simulink model "obsvsimulink"  (R2018b)
settings: Solver=VariableStepAuto  StartTime=0.0  StopTime=10  RelTol=1e-3
values from neighbouring files (symbols this model uses):
  A = [0 1 0 0 ... (first row only)    [kalman.m]    (also in lqr_controller.m; lqr_observare.m; state_space.m)
  B = [0 ... (first row only)    [kalman.m]    (also in lqr_controller.m; lqr_observare.m; state_space.m)
  C = [1 0 0 0;]    [kalman.m]    (also in lqr_controller.m = [1 0 0 0; lqr_observare.m = [1 0 0 0; state_space.m = [1 0 0 0)
  K_d = lqr(A,B,Q,R)    [lqr_observare.m]
  L_o = (place(A',C',E))'    [lqr_observare.m]
settings Model: Creator=SAFARBALI  LastModifiedBy=888
settings SFSimCC: SimUseLocalCustomCode=off
settings RTWCC: RTWUseLocalCustomCode=off
settings CodeAppCC: StateflowObjectComments=on

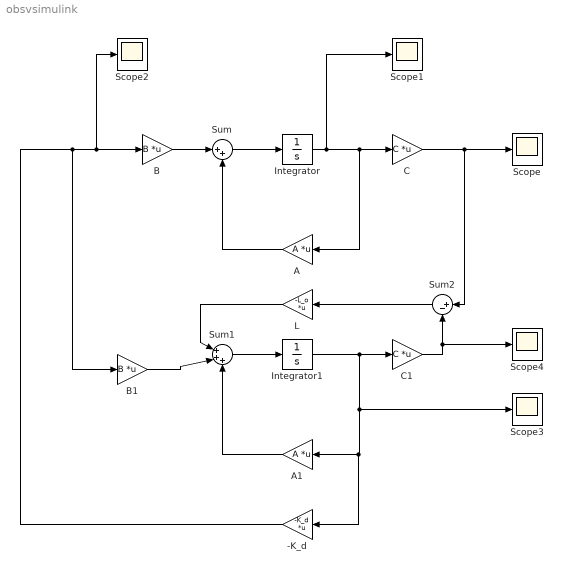
== system obsvsimulink ==
  -K_d : Gain  Gain=-K_d  Multiplication=Matrix(K*u)
  A : Gain  Gain=A  Multiplication=Matrix(K*u)
  A1 : Gain  Gain=A  Multiplication=Matrix(K*u)
  B : Gain  Gain=B  Multiplication=Matrix(K*u)
  B1 : Gain  Gain=B  Multiplication=Matrix(K*u)
  C : Gain  Gain=C  Multiplication=Matrix(K*u)
  C1 : Gain  Gain=C  Multiplication=Matrix(K*u)
  Integrator : Integrator  InitialCondition=[0;5;0;0]
  Integrator1 : Integrator  InitialCondition=[0;5;0;0]
  L : Gain  Gain=-L_o  Multiplication=Matrix(K*u)
  Scope{,1..4} (5 alike) : Scope
  Sum : Sum  Inputs=|++
  Sum1 : Sum  Inputs=|+++
  Sum2 : Sum  Inputs=|+-
  wires:
  Integrator/1 -> A/1, C/1, Scope1/1
  C/1 -> Sum2/1, Scope/1
  Sum/1 -> Integrator/1
  B/1 -> Sum/1
  A/1 -> Sum/2
  A1/1 -> Sum1/3
  B1/1 -> Sum1/2
  Sum1/1 -> Integrator1/1
  Integrator1/1 -> C1/1, -K_d/1, A1/1, Scope3/1
  C1/1 -> Scope4/1, Sum2/2
  Sum2/1 -> L/1
  L/1 -> Sum1/1
  -K_d/1 -> B1/1, Scope2/1, B/1
